simulink model "ErskineMultiDroneFormation"  (R2019b)
settings: Solver=FixedStepAuto  StartTime=0.0  StopTime=Tsim  FixedStep=sim_dt  RelTol=1e-3
values from neighbouring files (symbols this model uses):
  controller_rate = 25    [MultiQuadInit.m]
  drone_params = setDefaultDroneParams(nDrones)    [MultiQuadInit.m]    (also in SingleQuadInit.m = setDefaultDroneParams(1))
  dt_p = 0.1    [MultiQuadInit.m]
  edges = [1,2 ... (first row only)    [MultiQuadInit.m]
  g = 9.81    [MultiQuadInit.m]    (also in SingleQuadInit.m)
  N_p = 1    [MultiQuadInit.m]
  nDrones = 3    [MultiQuadInit.m]
  omega0 = zeros(3,nDrones)    [MultiQuadInit.m]    (also in SingleQuadInit.m = [0;0;0])
  p0 = 4*(rand(3,nDrones) - [0.5;0.5;0])    [MultiQuadInit.m]    (also in SingleQuadInit.m = 4*(rand(3, 1) - [0.5;0.5;0]))
  q0 = zeros(4,nDrones); q0(1,:) = ones(1,nDrones)    [MultiQuadInit.m]    (also in SingleQuadInit.m = [1;0;0;0])
  sim_dt = 0.005    [MultiQuadInit.m]    (also in SingleQuadInit.m)
  v0 = zeros(3, nDrones)    [MultiQuadInit.m]    (also in SingleQuadInit.m = [0;0;0])
undefined symbols (not defined in the file or in its folder): camera_noise
libraries: vrlib x6
(part 1 of 2)
settings Model: Creator=julian  LastModifiedBy=julian

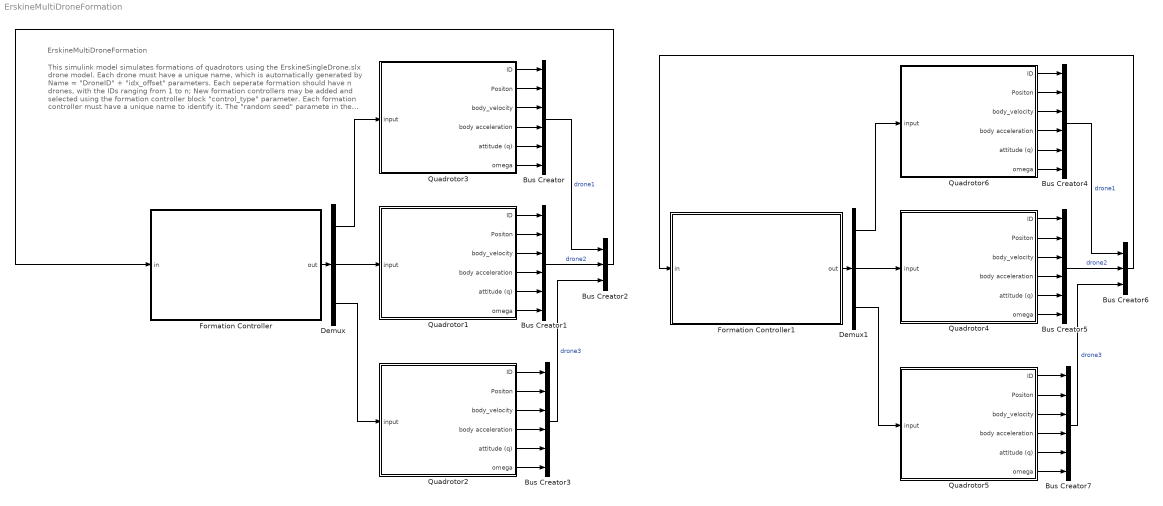
== system ErskineMultiDroneFormation ==
  note: This simulink model simulates formations of quadrotors using the
      | ErskineSingleDrone.slx drone model.  Each drone must have a unique name,
      | which is automatically generated by Name = "DroneID" + "idx_offset" parameters.
      | Each seperate formation should have n drones, with the IDs ranging from 1 to n;
      |
      | New formation controllers may be added and selected using the formation
      | controller block "control_type" parameter. Each formation controller must have a
      | unique name to identify it. The "random seed" paramete in the formation control block sets the random noise seed for the controller measurements.
      |
      | Initial conditions, parameters, and the FormationStateBus must be generated for n drones (see initialization script)
  note: ErskineMultiDroneFormation
  "  Quadrotor1" : Subsystem  mask{control_type_param=2: Body Velocity + Yawrate, DroneID=2, DroneName=Drone2, idx_offset=0}
      mask prompts: control_type_param "Controller type"; DroneName "Drone Name"; idx_offset "Index Offset"
      mask TypeOptions control_type_param: 1: Position + Yaw | 2: Body Velocity + Yawrate | 3: Body Acceleration + Yawrate | 4: Thrust + Attitude | 5: Thrust + Body Rate | 6: Body Wrench
      mask TypeOptions DroneID: 1 | 2 | 3 | 4 | 5 | 6 | 7 | 8 | 9
      mask Callback DroneID:
      | ID = get_param(gcb,'DroneID');
      | offset = get_param(gcb,'idx_offset');
      | if ischar(ID)
      |   ID = str2num(ID);
      | end
      | if ischar(offset)
      |   offset = str2num(offset);
      | end
      | nameID = ID + offset;
      | set_param(gcb,'DroneName',["Drone"+num2str(nameID)]);
      mask Callback DroneName: set_param([gcb,'/To Workspace'],'VariableName',[get_param(gcb,'DroneName')]);
      mask Callback idx_offset:
      | ID = get_param(gcb,'DroneID');
      | offset = get_param(gcb,'idx_offset');
      | if ischar(ID)
      |   ID = str2num(ID);
      | end
      | if ischar(offset)
      |   offset = str2num(offset);
      | end
      | nameID = ID + offset;
      | set_param(gcb,'DroneName',["Drone"+num2str(nameID)]);
      mask DialogControl Control4 Prompt: click to choose controller
      mask Display:
      | image('Format/drone_image.png'); % Use "Edit Image" on toolstrip to change.
      | Name = get_param(gcb,'DroneName');
      | ID = get_param(gcb,'DroneID');
      | C_mode = get_param(gcb,'control_type_param');
      | C_mode(1:2) = [];
      | color('red')
      | ID = "ID = "+ID;
      | color('red')
      | text(0.5, 0.25, Name, 'horizontalAlignment', 'center')
      | color('red')
      | text(0.5, 0.15, ID, 'horizontalAlignment', 'center')
      | color('blue');
      | text(0.5, 0.05, C_mode, 'horizontalAlignment', 'center')
  "  Quadrotor2" : Subsystem  mask{control_type_param=2: Body Velocity + Yawrate, DroneID=3, DroneName=Drone3, idx_offset=0}
      mask prompts: control_type_param "Controller type"; DroneName "Drone Name"; idx_offset "Index Offset"
      mask TypeOptions control_type_param: 1: Position + Yaw | 2: Body Velocity + Yawrate | 3: Body Acceleration + Yawrate | 4: Thrust + Attitude | 5: Thrust + Body Rate | 6: Body Wrench
      mask TypeOptions DroneID: 1 | 2 | 3 | 4 | 5 | 6 | 7 | 8 | 9
      mask Callback DroneID:
      | ID = get_param(gcb,'DroneID');
      | offset = get_param(gcb,'idx_offset');
      | if ischar(ID)
      |   ID = str2num(ID);
      | end
      | if ischar(offset)
      |   offset = str2num(offset);
      | end
      | nameID = ID + offset;
      | set_param(gcb,'DroneName',["Drone"+num2str(nameID)]);
      mask Callback DroneName: set_param([gcb,'/To Workspace'],'VariableName',[get_param(gcb,'DroneName')]);
      mask Callback idx_offset:
      | ID = get_param(gcb,'DroneID');
      | offset = get_param(gcb,'idx_offset');
      | if ischar(ID)
      |   ID = str2num(ID);
      | end
      | if ischar(offset)
      |   offset = str2num(offset);
      | end
      | nameID = ID + offset;
      | set_param(gcb,'DroneName',["Drone"+num2str(nameID)]);
      mask DialogControl Control4 Prompt: click to choose controller
      mask Display:
      | image('Format/drone_image.png'); % Use "Edit Image" on toolstrip to change.
      | Name = get_param(gcb,'DroneName');
      | ID = get_param(gcb,'DroneID');
      | C_mode = get_param(gcb,'control_type_param');
      | C_mode(1:2) = [];
      | color('red')
      | ID = "ID = "+ID;
      | color('red')
      | text(0.5, 0.25, Name, 'horizontalAlignment', 'center')
      | color('red')
      | text(0.5, 0.15, ID, 'horizontalAlignment', 'center')
      | color('blue');
      | text(0.5, 0.05, C_mode, 'horizontalAlignment', 'center')
  "  Quadrotor3" : Subsystem  mask{control_type_param=2: Body Velocity + Yawrate, DroneID=1, DroneName=Drone1, idx_offset=0}
      mask prompts: control_type_param "Controller type"; DroneName "Drone Name"; idx_offset "Index Offset"
      mask TypeOptions control_type_param: 1: Position + Yaw | 2: Body Velocity + Yawrate | 3: Body Acceleration + Yawrate | 4: Thrust + Attitude | 5: Thrust + Body Rate | 6: Body Wrench
      mask TypeOptions DroneID: 1 | 2 | 3 | 4 | 5 | 6 | 7 | 8 | 9
      mask Callback DroneID:
      | ID = get_param(gcb,'DroneID');
      | offset = get_param(gcb,'idx_offset');
      | if ischar(ID)
      |   ID = str2num(ID);
      | end
      | if ischar(offset)
      |   offset = str2num(offset);
      | end
      | nameID = ID + offset;
      | set_param(gcb,'DroneName',["Drone"+num2str(nameID)]);
      mask Callback DroneName: set_param([gcb,'/To Workspace'],'VariableName',[get_param(gcb,'DroneName')]);
      mask Callback idx_offset:
      | ID = get_param(gcb,'DroneID');
      | offset = get_param(gcb,'idx_offset');
      | if ischar(ID)
      |   ID = str2num(ID);
      | end
      | if ischar(offset)
      |   offset = str2num(offset);
      | end
      | nameID = ID + offset;
      | set_param(gcb,'DroneName',["Drone"+num2str(nameID)]);
      mask DialogControl Control4 Prompt: click to choose controller
      mask Display:
      | image('Format/drone_image.png'); % Use "Edit Image" on toolstrip to change.
      | Name = get_param(gcb,'DroneName');
      | ID = get_param(gcb,'DroneID');
      | C_mode = get_param(gcb,'control_type_param');
      | C_mode(1:2) = [];
      | color('red')
      | ID = "ID = "+ID;
      | color('red')
      | text(0.5, 0.25, Name, 'horizontalAlignment', 'center')
      | color('red')
      | text(0.5, 0.15, ID, 'horizontalAlignment', 'center')
      | color('blue');
      | text(0.5, 0.05, C_mode, 'horizontalAlignment', 'center')
  "  Quadrotor4" : Subsystem  mask{control_type_param=2: Body Velocity + Yawrate, DroneID=2, DroneName=Drone5, idx_offset=3}
      mask prompts: control_type_param "Controller type"; DroneName "Drone Name"; idx_offset "Index Offset"
      mask TypeOptions control_type_param: 1: Position + Yaw | 2: Body Velocity + Yawrate | 3: Body Acceleration + Yawrate | 4: Thrust + Attitude | 5: Thrust + Body Rate | 6: Body Wrench
      mask TypeOptions DroneID: 1 | 2 | 3 | 4 | 5 | 6 | 7 | 8 | 9
      mask Callback DroneID:
      | ID = get_param(gcb,'DroneID');
      | offset = get_param(gcb,'idx_offset');
      | if ischar(ID)
      |   ID = str2num(ID);
      | end
      | if ischar(offset)
      |   offset = str2num(offset);
      | end
      | nameID = ID + offset;
      | set_param(gcb,'DroneName',["Drone"+num2str(nameID)]);
      mask Callback DroneName: set_param([gcb,'/To Workspace'],'VariableName',[get_param(gcb,'DroneName')]);
      mask Callback idx_offset:
      | ID = get_param(gcb,'DroneID');
      | offset = get_param(gcb,'idx_offset');
      | if ischar(ID)
      |   ID = str2num(ID);
      | end
      | if ischar(offset)
      |   offset = str2num(offset);
      | end
      | nameID = ID + offset;
      | set_param(gcb,'DroneName',["Drone"+num2str(nameID)]);
      mask DialogControl Control4 Prompt: click to choose controller
      mask Display:
      | image('Format/drone_image.png'); % Use "Edit Image" on toolstrip to change.
      | Name = get_param(gcb,'DroneName');
      | ID = get_param(gcb,'DroneID');
      | C_mode = get_param(gcb,'control_type_param');
      | C_mode(1:2) = [];
      | color('red')
      | ID = "ID = "+ID;
      | color('red')
      | text(0.5, 0.25, Name, 'horizontalAlignment', 'center')
      | color('red')
      | text(0.5, 0.15, ID, 'horizontalAlignment', 'center')
      | color('blue');
      | text(0.5, 0.05, C_mode, 'horizontalAlignment', 'center')
  "  Quadrotor5" : Subsystem  mask{control_type_param=2: Body Velocity + Yawrate, DroneID=3, DroneName=Drone6, idx_offset=3}
      mask prompts: control_type_param "Controller type"; DroneName "Drone Name"; idx_offset "Index Offset"
      mask TypeOptions control_type_param: 1: Position + Yaw | 2: Body Velocity + Yawrate | 3: Body Acceleration + Yawrate | 4: Thrust + Attitude | 5: Thrust + Body Rate | 6: Body Wrench
      mask TypeOptions DroneID: 1 | 2 | 3 | 4 | 5 | 6 | 7 | 8 | 9
      mask Callback DroneID:
      | ID = get_param(gcb,'DroneID');
      | offset = get_param(gcb,'idx_offset');
      | if ischar(ID)
      |   ID = str2num(ID);
      | end
      | if ischar(offset)
      |   offset = str2num(offset);
      | end
      | nameID = ID + offset;
      | set_param(gcb,'DroneName',["Drone"+num2str(nameID)]);
      mask Callback DroneName: set_param([gcb,'/To Workspace'],'VariableName',[get_param(gcb,'DroneName')]);
      mask Callback idx_offset:
      | ID = get_param(gcb,'DroneID');
      | offset = get_param(gcb,'idx_offset');
      | if ischar(ID)
      |   ID = str2num(ID);
      | end
      | if ischar(offset)
      |   offset = str2num(offset);
      | end
      | nameID = ID + offset;
      | set_param(gcb,'DroneName',["Drone"+num2str(nameID)]);
      mask DialogControl Control4 Prompt: click to choose controller
      mask Display:
      | image('Format/drone_image.png'); % Use "Edit Image" on toolstrip to change.
      | Name = get_param(gcb,'DroneName');
      | ID = get_param(gcb,'DroneID');
      | C_mode = get_param(gcb,'control_type_param');
      | C_mode(1:2) = [];
      | color('red')
      | ID = "ID = "+ID;
      | color('red')
      | text(0.5, 0.25, Name, 'horizontalAlignment', 'center')
      | color('red')
      | text(0.5, 0.15, ID, 'horizontalAlignment', 'center')
      | color('blue');
      | text(0.5, 0.05, C_mode, 'horizontalAlignment', 'center')
  "  Quadrotor6" : Subsystem  mask{control_type_param=2: Body Velocity + Yawrate, DroneID=1, DroneName=Drone4, idx_offset=3}
      mask prompts: control_type_param "Controller type"; DroneName "Drone Name"; idx_offset "Index Offset"
      mask TypeOptions control_type_param: 1: Position + Yaw | 2: Body Velocity + Yawrate | 3: Body Acceleration + Yawrate | 4: Thrust + Attitude | 5: Thrust + Body Rate | 6: Body Wrench
      mask TypeOptions DroneID: 1 | 2 | 3 | 4 | 5 | 6 | 7 | 8 | 9
      mask Callback DroneID:
      | ID = get_param(gcb,'DroneID');
      | offset = get_param(gcb,'idx_offset');
      | if ischar(ID)
      |   ID = str2num(ID);
      | end
      | if ischar(offset)
      |   offset = str2num(offset);
      | end
      | nameID = ID + offset;
      | set_param(gcb,'DroneName',["Drone"+num2str(nameID)]);
      mask Callback DroneName: set_param([gcb,'/To Workspace'],'VariableName',[get_param(gcb,'DroneName')]);
      mask Callback idx_offset:
      | ID = get_param(gcb,'DroneID');
      | offset = get_param(gcb,'idx_offset');
      | if ischar(ID)
      |   ID = str2num(ID);
      | end
      | if ischar(offset)
      |   offset = str2num(offset);
      | end
      | nameID = ID + offset;
      | set_param(gcb,'DroneName',["Drone"+num2str(nameID)]);
      mask DialogControl Control4 Prompt: click to choose controller
      mask Display:
      | image('Format/drone_image.png'); % Use "Edit Image" on toolstrip to change.
      | Name = get_param(gcb,'DroneName');
      | ID = get_param(gcb,'DroneID');
      | C_mode = get_param(gcb,'control_type_param');
      | C_mode(1:2) = [];
      | color('red')
      | ID = "ID = "+ID;
      | color('red')
      | text(0.5, 0.25, Name, 'horizontalAlignment', 'center')
      | color('red')
      | text(0.5, 0.15, ID, 'horizontalAlignment', 'center')
      | color('blue');
      | text(0.5, 0.05, C_mode, 'horizontalAlignment', 'center')
  Bus Creator{,1,3..5,7} (6 alike) : BusCreator  Inputs=6  OutDataTypeStr=Bus: DroneStateBus
      settings: InheritFromInputs=off
  Bus Creator2 : BusCreator  Inputs=3  OutDataTypeStr=Bus: FormationStateBus  NonVirtualBus=on
      settings: InheritFromInputs=off
  Bus Creator6 : BusCreator  Inputs=3  OutDataTypeStr=Bus: FormationStateBus  NonVirtualBus=on
      settings: InheritFromInputs=off
  Demux : Demux  Outputs=3
  Demux1 : Demux  Outputs=3
  Formation Controller : Subsystem  mask(FormationController){seed_type=Random, rng_seed=9730, control_type=1: Gradient, out_name=Gradient}
      mask prompts: seed_type "Random Seed"; rng_seed "Custom Seed"; control_type "Formation Control Type"; out_name "Out Name"
      mask TypeOptions seed_type: Random | Custom
      mask Callback seed_type:
      | box_A = get_param(gcb, 'seed_type');
      | m = Simulink.Mask.get(gcb);
      | box_B = m.getParameter('rng_seed');
      | 
      | if strcmp(box_A, 'Random')
      |     seed = randi([1,10000]);
      |     set_param(gcb,'rng_seed', num2str(seed));
      |     box_B.Enabled = 'off';
      | else
      |     box_B.Enabled = 'on';
      | end
      mask TypeOptions control_type: 1: Gradient | 2: Faster Gradient
      mask Callback out_name: set_param([gcb,'/To Workspace'],'VariableName',[get_param(gcb,'out_name')]);
      mask Display:
      | image('$imagefile'); % Use "Edit Image" on toolstrip to change.
      | type = get_param(gcb,'control_type');
      | color('red')
      | text(0.5, 0.25, type, 'horizontalAlignment', 'center')
  Formation Controller1 : Subsystem  mask(FormationController){seed_type=Random, rng_seed=5186, control_type=2: Faster Gradient, out_name=PoorlyTunedGradient}
      mask prompts: seed_type "Random Seed"; rng_seed "Custom Seed"; control_type "Formation Control Type"; out_name "Out Name"
      mask TypeOptions seed_type: Random | Custom
      mask Callback seed_type:
      | box_A = get_param(gcb, 'seed_type');
      | m = Simulink.Mask.get(gcb);
      | box_B = m.getParameter('rng_seed');
      | 
      | if strcmp(box_A, 'Random')
      |     seed = randi([1,10000]);
      |     set_param(gcb,'rng_seed', num2str(seed));
      |     box_B.Enabled = 'off';
      | else
      |     box_B.Enabled = 'on';
      | end
      mask TypeOptions control_type: 1: Gradient | 2: Faster Gradient
      mask Callback out_name: set_param([gcb,'/To Workspace'],'VariableName',[get_param(gcb,'out_name')]);
      mask Display:
      | image('$imagefile'); % Use "Edit Image" on toolstrip to change.
      | type = get_param(gcb,'control_type');
      | color('red')
      | text(0.5, 0.25, type, 'horizontalAlignment', 'center')
  wires:
  "  Quadrotor3"/6(omega) -> Bus Creator/6
  "  Quadrotor3"/5(attitude (q)) -> Bus Creator/5
  "  Quadrotor3"/4(body acceleration) -> Bus Creator/4
  "  Quadrotor3"/3(body_velocity) -> Bus Creator/3
  "  Quadrotor3"/2(Positon) -> Bus Creator/2
  "  Quadrotor3"/1(ID) -> Bus Creator/1
  "  Quadrotor1"/1(ID) -> Bus Creator1/1
  "  Quadrotor1"/2(Positon) -> Bus Creator1/2
  "  Quadrotor1"/3(body_velocity) -> Bus Creator1/3
  "  Quadrotor1"/4(body acceleration) -> Bus Creator1/4
  "  Quadrotor1"/5(attitude (q)) -> Bus Creator1/5
  "  Quadrotor1"/6(omega) -> Bus Creator1/6
  Bus Creator/1 -> Bus Creator2/1  "drone1"
  Bus Creator1/1 -> Bus Creator2/2  "drone2"
  Bus Creator2/1 -> Formation Controller/1(in)
  Formation Controller/1(out) -> Demux/1
  "  Quadrotor2"/1(ID) -> Bus Creator3/1
  "  Quadrotor2"/2(Positon) -> Bus Creator3/2
  "  Quadrotor2"/3(body_velocity) -> Bus Creator3/3
  "  Quadrotor2"/4(body acceleration) -> Bus Creator3/4
  "  Quadrotor2"/5(attitude (q)) -> Bus Creator3/5
  "  Quadrotor2"/6(omega) -> Bus Creator3/6
  Bus Creator3/1 -> Bus Creator2/3  "drone3"
  Demux/1 -> "  Quadrotor3"/1(input)
  Demux/2 -> "  Quadrotor1"/1(input)
  Demux/3 -> "  Quadrotor2"/1(input)
  Demux1/2 -> "  Quadrotor4"/1(input)
  "  Quadrotor5"/3(body_velocity) -> Bus Creator7/3
  "  Quadrotor6"/1(ID) -> Bus Creator4/1
  "  Quadrotor6"/4(body acceleration) -> Bus Creator4/4
  "  Quadrotor4"/1(ID) -> Bus Creator5/1
  "  Quadrotor4"/2(Positon) -> Bus Creator5/2
  "  Quadrotor6"/2(Positon) -> Bus Creator4/2
  "  Quadrotor4"/3(body_velocity) -> Bus Creator5/3
  "  Quadrotor4"/4(body acceleration) -> Bus Creator5/4
  "  Quadrotor4"/5(attitude (q)) -> Bus Creator5/5
  "  Quadrotor6"/6(omega) -> Bus Creator4/6
  Bus Creator6/1 -> Formation Controller1/1(in)
  "  Quadrotor5"/4(body acceleration) -> Bus Creator7/4
  Bus Creator4/1 -> Bus Creator6/1  "drone1"
  "  Quadrotor4"/6(omega) -> Bus Creator5/6
  Bus Creator5/1 -> Bus Creator6/2  "drone2"
  "  Quadrotor5"/2(Positon) -> Bus Creator7/2
  Demux1/1 -> "  Quadrotor6"/1(input)
  Bus Creator7/1 -> Bus Creator6/3  "drone3"
  Formation Controller1/1(out) -> Demux1/1
  "  Quadrotor5"/6(omega) -> Bus Creator7/6
  "  Quadrotor6"/5(attitude (q)) -> Bus Creator4/5
  Demux1/3 -> "  Quadrotor5"/1(input)
  "  Quadrotor6"/3(body_velocity) -> Bus Creator4/3
  "  Quadrotor5"/5(attitude (q)) -> Bus Creator7/5
  "  Quadrotor5"/1(ID) -> Bus Creator7/1

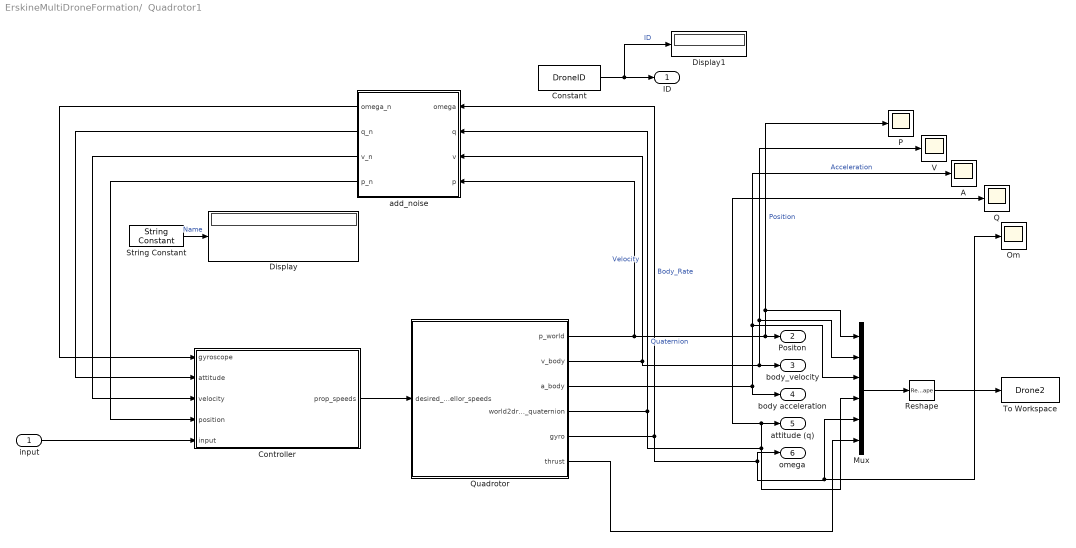
== system ErskineMultiDroneFormation/  Quadrotor1 ==
  input : Inport
  A : Scope
  Constant : Constant  Value=DroneID
  Controller : Subsystem
      mask Display: image('Format/flightController.png'); % Use "Edit Image" on toolstrip to change.
  Display : Display
  Display1 : Display
  Mux : Mux  Inputs=6
  Om : Scope
  P : Scope
  Q : Scope
  Quadrotor : Subsystem
      mask Display: image('droneHardware.jpeg'); % Use "Edit Image" on toolstrip to change.
  Reshape : Reshape
  String Constant : StringConstant  String=DroneName
  To Workspace : ToWorkspace  VariableName=Drone2  SaveFormat=Timeseries  SampleTime=-1
  V : Scope
  add_noise : MATLAB Function  TreatAsAtomicUnit=on
  ID : Outport
  Positon : Outport  Port=2
  body_velocity : Outport  Port=3
  body acceleration : Outport  Port=4
  attitude (q) : Outport  Port=5
  omega : Outport  Port=6
  wires:
  Quadrotor/5(gyro) -> Om/1, Mux/5, omega/1, add_noise/1(omega)  "Body_Rate"
  Quadrotor/1(p_world) -> add_noise/4(p), P/1, Mux/1, Positon/1  "Position"
  Quadrotor/3(a_body) -> body acceleration/1, A/1, Mux/3  "Acceleration"
  Quadrotor/4(world2drone_quaternion) -> Q/1, attitude (q)/1, Mux/4, add_noise/2(q)  "Quaternion"
  Mux/1 -> Reshape/1
  Quadrotor/2(v_body) -> V/1, Mux/2, body_velocity/1, add_noise/3(v)  "Velocity"
  Quadrotor/6(thrust) -> Mux/6
  String Constant/1 -> Display/1  "Name"
  Constant/1 -> Display1/1, ID/1  "ID"
  Reshape/1 -> To Workspace/1
  add_noise/1(omega_n) -> Controller/1(gyroscope)
  add_noise/2(q_n) -> Controller/2(attitude)
  add_noise/3(v_n) -> Controller/3(velocity)
  add_noise/4(p_n) -> Controller/4(position)
  input/1 -> Controller/5(input)
  Controller/1(prop_speeds) -> Quadrotor/1(desired_propellor_speeds)

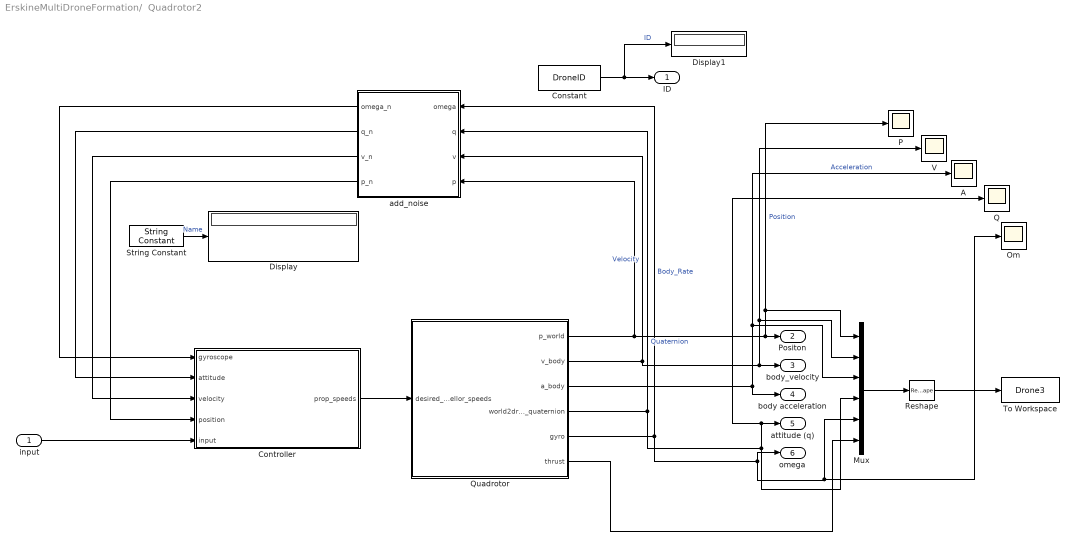
== system ErskineMultiDroneFormation/  Quadrotor2 ==
  input : Inport
  A : Scope
  Constant : Constant  Value=DroneID
  Controller : Subsystem
      mask Display: image('Format/flightController.png'); % Use "Edit Image" on toolstrip to change.
  Display : Display
  Display1 : Display
  Mux : Mux  Inputs=6
  Om : Scope
  P : Scope
  Q : Scope
  Quadrotor : Subsystem
      mask Display: image('droneHardware.jpeg'); % Use "Edit Image" on toolstrip to change.
  Reshape : Reshape
  String Constant : StringConstant  String=DroneName
  To Workspace : ToWorkspace  VariableName=Drone3  SaveFormat=Timeseries  SampleTime=-1
  V : Scope
  add_noise : MATLAB Function  TreatAsAtomicUnit=on
  ID : Outport
  Positon : Outport  Port=2
  body_velocity : Outport  Port=3
  body acceleration : Outport  Port=4
  attitude (q) : Outport  Port=5
  omega : Outport  Port=6
  wires:
  Quadrotor/5(gyro) -> Om/1, Mux/5, omega/1, add_noise/1(omega)  "Body_Rate"
  Quadrotor/1(p_world) -> add_noise/4(p), P/1, Mux/1, Positon/1  "Position"
  Quadrotor/3(a_body) -> body acceleration/1, A/1, Mux/3  "Acceleration"
  Quadrotor/4(world2drone_quaternion) -> Q/1, attitude (q)/1, Mux/4, add_noise/2(q)  "Quaternion"
  Mux/1 -> Reshape/1
  Quadrotor/2(v_body) -> V/1, Mux/2, body_velocity/1, add_noise/3(v)  "Velocity"
  Quadrotor/6(thrust) -> Mux/6
  String Constant/1 -> Display/1  "Name"
  Constant/1 -> Display1/1, ID/1  "ID"
  Reshape/1 -> To Workspace/1
  add_noise/1(omega_n) -> Controller/1(gyroscope)
  add_noise/2(q_n) -> Controller/2(attitude)
  add_noise/3(v_n) -> Controller/3(velocity)
  add_noise/4(p_n) -> Controller/4(position)
  input/1 -> Controller/5(input)
  Controller/1(prop_speeds) -> Quadrotor/1(desired_propellor_speeds)

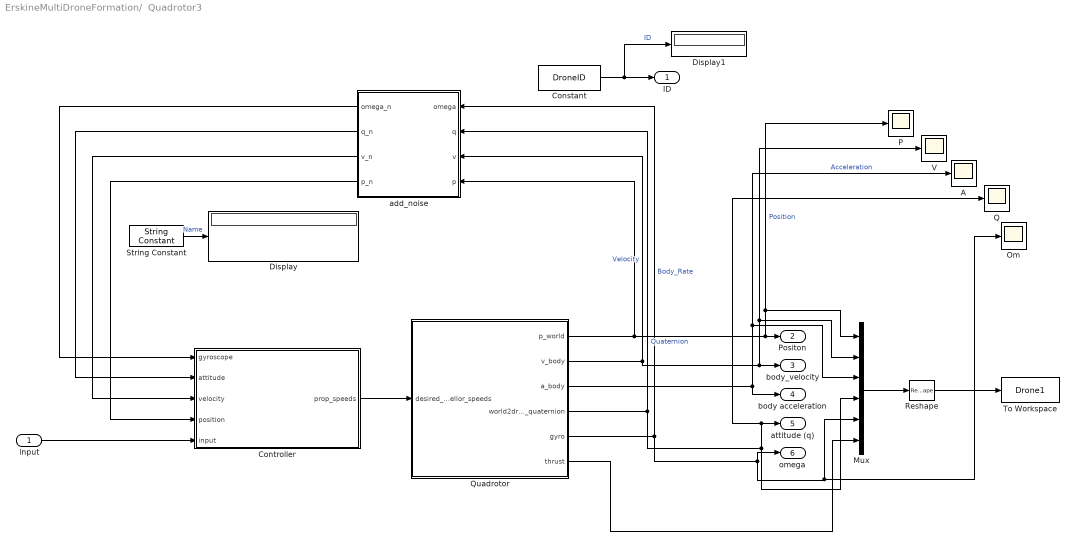
== system ErskineMultiDroneFormation/  Quadrotor3 ==
  input : Inport
  A : Scope
  Constant : Constant  Value=DroneID
  Controller : Subsystem
      mask Display: image('Format/flightController.png'); % Use "Edit Image" on toolstrip to change.
  Display : Display
  Display1 : Display
  Mux : Mux  Inputs=6
  Om : Scope
  P : Scope
  Q : Scope
  Quadrotor : Subsystem
      mask Display: image('droneHardware.jpeg'); % Use "Edit Image" on toolstrip to change.
  Reshape : Reshape
  String Constant : StringConstant  String=DroneName
  To Workspace : ToWorkspace  VariableName=Drone1  SaveFormat=Timeseries  SampleTime=-1
  V : Scope
  add_noise : MATLAB Function  TreatAsAtomicUnit=on
  ID : Outport
  Positon : Outport  Port=2
  body_velocity : Outport  Port=3
  body acceleration : Outport  Port=4
  attitude (q) : Outport  Port=5
  omega : Outport  Port=6
  wires:
  Quadrotor/5(gyro) -> Om/1, Mux/5, omega/1, add_noise/1(omega)  "Body_Rate"
  Quadrotor/1(p_world) -> add_noise/4(p), P/1, Mux/1, Positon/1  "Position"
  Quadrotor/3(a_body) -> body acceleration/1, A/1, Mux/3  "Acceleration"
  Quadrotor/4(world2drone_quaternion) -> Q/1, attitude (q)/1, Mux/4, add_noise/2(q)  "Quaternion"
  Mux/1 -> Reshape/1
  Quadrotor/2(v_body) -> V/1, Mux/2, body_velocity/1, add_noise/3(v)  "Velocity"
  Quadrotor/6(thrust) -> Mux/6
  String Constant/1 -> Display/1  "Name"
  Constant/1 -> Display1/1, ID/1  "ID"
  Reshape/1 -> To Workspace/1
  add_noise/1(omega_n) -> Controller/1(gyroscope)
  add_noise/2(q_n) -> Controller/2(attitude)
  add_noise/3(v_n) -> Controller/3(velocity)
  add_noise/4(p_n) -> Controller/4(position)
  input/1 -> Controller/5(input)
  Controller/1(prop_speeds) -> Quadrotor/1(desired_propellor_speeds)

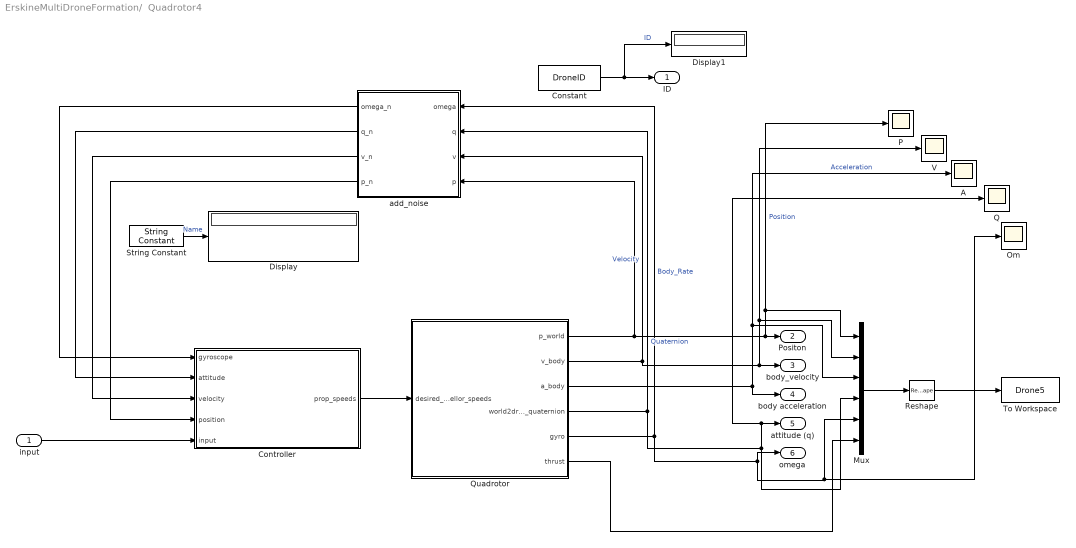
== system ErskineMultiDroneFormation/  Quadrotor4 ==
  input : Inport
  A : Scope
  Constant : Constant  Value=DroneID
  Controller : Subsystem
      mask Display: image('Format/flightController.png'); % Use "Edit Image" on toolstrip to change.
  Display : Display
  Display1 : Display
  Mux : Mux  Inputs=6
  Om : Scope
  P : Scope
  Q : Scope
  Quadrotor : Subsystem
      mask Display: image('droneHardware.jpeg'); % Use "Edit Image" on toolstrip to change.
  Reshape : Reshape
  String Constant : StringConstant  String=DroneName
  To Workspace : ToWorkspace  VariableName=Drone5  SaveFormat=Timeseries  SampleTime=-1
  V : Scope
  add_noise : MATLAB Function  TreatAsAtomicUnit=on
  ID : Outport
  Positon : Outport  Port=2
  body_velocity : Outport  Port=3
  body acceleration : Outport  Port=4
  attitude (q) : Outport  Port=5
  omega : Outport  Port=6
  wires:
  Quadrotor/5(gyro) -> Om/1, Mux/5, omega/1, add_noise/1(omega)  "Body_Rate"
  Quadrotor/1(p_world) -> add_noise/4(p), P/1, Mux/1, Positon/1  "Position"
  Quadrotor/3(a_body) -> body acceleration/1, A/1, Mux/3  "Acceleration"
  Quadrotor/4(world2drone_quaternion) -> Q/1, attitude (q)/1, Mux/4, add_noise/2(q)  "Quaternion"
  Mux/1 -> Reshape/1
  Quadrotor/2(v_body) -> V/1, Mux/2, body_velocity/1, add_noise/3(v)  "Velocity"
  Quadrotor/6(thrust) -> Mux/6
  String Constant/1 -> Display/1  "Name"
  Constant/1 -> Display1/1, ID/1  "ID"
  Reshape/1 -> To Workspace/1
  add_noise/1(omega_n) -> Controller/1(gyroscope)
  add_noise/2(q_n) -> Controller/2(attitude)
  add_noise/3(v_n) -> Controller/3(velocity)
  add_noise/4(p_n) -> Controller/4(position)
  input/1 -> Controller/5(input)
  Controller/1(prop_speeds) -> Quadrotor/1(desired_propellor_speeds)

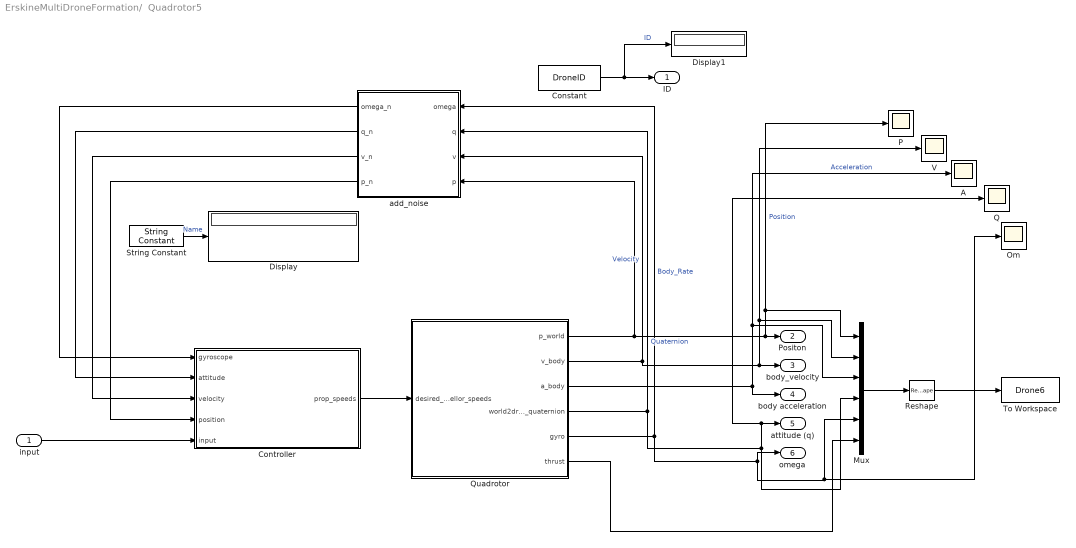
== system ErskineMultiDroneFormation/  Quadrotor5 ==
  input : Inport
  A : Scope
  Constant : Constant  Value=DroneID
  Controller : Subsystem
      mask Display: image('Format/flightController.png'); % Use "Edit Image" on toolstrip to change.
  Display : Display
  Display1 : Display
  Mux : Mux  Inputs=6
  Om : Scope
  P : Scope
  Q : Scope
  Quadrotor : Subsystem
      mask Display: image('droneHardware.jpeg'); % Use "Edit Image" on toolstrip to change.
  Reshape : Reshape
  String Constant : StringConstant  String=DroneName
  To Workspace : ToWorkspace  VariableName=Drone6  SaveFormat=Timeseries  SampleTime=-1
  V : Scope
  add_noise : MATLAB Function  TreatAsAtomicUnit=on
  ID : Outport
  Positon : Outport  Port=2
  body_velocity : Outport  Port=3
  body acceleration : Outport  Port=4
  attitude (q) : Outport  Port=5
  omega : Outport  Port=6
  wires:
  Quadrotor/5(gyro) -> Om/1, Mux/5, omega/1, add_noise/1(omega)  "Body_Rate"
  Quadrotor/1(p_world) -> add_noise/4(p), P/1, Mux/1, Positon/1  "Position"
  Quadrotor/3(a_body) -> body acceleration/1, A/1, Mux/3  "Acceleration"
  Quadrotor/4(world2drone_quaternion) -> Q/1, attitude (q)/1, Mux/4, add_noise/2(q)  "Quaternion"
  Mux/1 -> Reshape/1
  Quadrotor/2(v_body) -> V/1, Mux/2, body_velocity/1, add_noise/3(v)  "Velocity"
  Quadrotor/6(thrust) -> Mux/6
  String Constant/1 -> Display/1  "Name"
  Constant/1 -> Display1/1, ID/1  "ID"
  Reshape/1 -> To Workspace/1
  add_noise/1(omega_n) -> Controller/1(gyroscope)
  add_noise/2(q_n) -> Controller/2(attitude)
  add_noise/3(v_n) -> Controller/3(velocity)
  add_noise/4(p_n) -> Controller/4(position)
  input/1 -> Controller/5(input)
  Controller/1(prop_speeds) -> Quadrotor/1(desired_propellor_speeds)

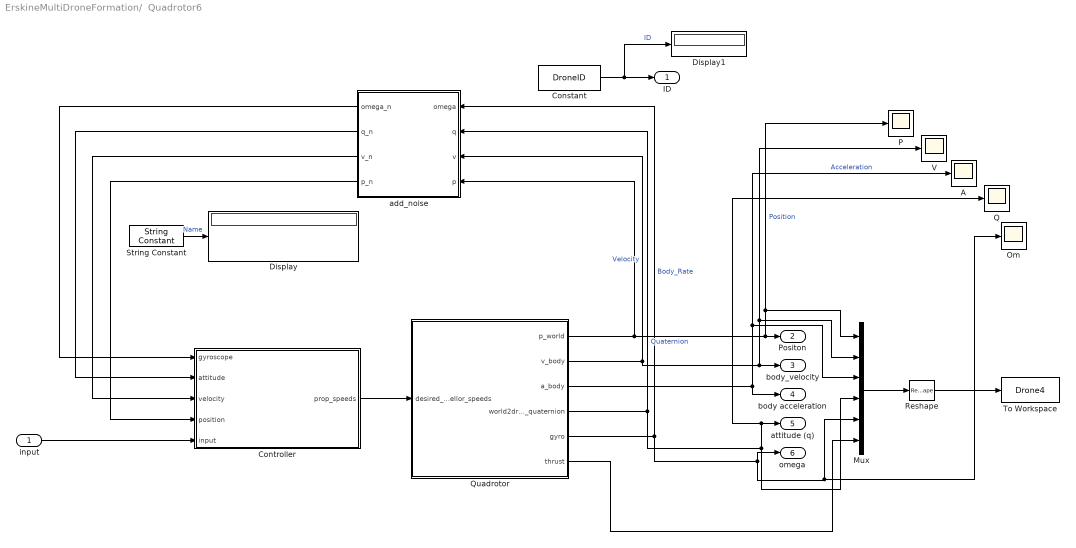
== system ErskineMultiDroneFormation/  Quadrotor6 ==
  input : Inport
  A : Scope
  Constant : Constant  Value=DroneID
  Controller : Subsystem
      mask Display: image('Format/flightController.png'); % Use "Edit Image" on toolstrip to change.
  Display : Display
  Display1 : Display
  Mux : Mux  Inputs=6
  Om : Scope
  P : Scope
  Q : Scope
  Quadrotor : Subsystem
      mask Display: image('droneHardware.jpeg'); % Use "Edit Image" on toolstrip to change.
  Reshape : Reshape
  String Constant : StringConstant  String=DroneName
  To Workspace : ToWorkspace  VariableName=Drone4  SaveFormat=Timeseries  SampleTime=-1
  V : Scope
  add_noise : MATLAB Function  TreatAsAtomicUnit=on
  ID : Outport
  Positon : Outport  Port=2
  body_velocity : Outport  Port=3
  body acceleration : Outport  Port=4
  attitude (q) : Outport  Port=5
  omega : Outport  Port=6
  wires:
  Quadrotor/5(gyro) -> Om/1, Mux/5, omega/1, add_noise/1(omega)  "Body_Rate"
  Quadrotor/1(p_world) -> add_noise/4(p), P/1, Mux/1, Positon/1  "Position"
  Quadrotor/3(a_body) -> body acceleration/1, A/1, Mux/3  "Acceleration"
  Quadrotor/4(world2drone_quaternion) -> Q/1, attitude (q)/1, Mux/4, add_noise/2(q)  "Quaternion"
  Mux/1 -> Reshape/1
  Quadrotor/2(v_body) -> V/1, Mux/2, body_velocity/1, add_noise/3(v)  "Velocity"
  Quadrotor/6(thrust) -> Mux/6
  String Constant/1 -> Display/1  "Name"
  Constant/1 -> Display1/1, ID/1  "ID"
  Reshape/1 -> To Workspace/1
  add_noise/1(omega_n) -> Controller/1(gyroscope)
  add_noise/2(q_n) -> Controller/2(attitude)
  add_noise/3(v_n) -> Controller/3(velocity)
  add_noise/4(p_n) -> Controller/4(position)
  input/1 -> Controller/5(input)
  Controller/1(prop_speeds) -> Quadrotor/1(desired_propellor_speeds)

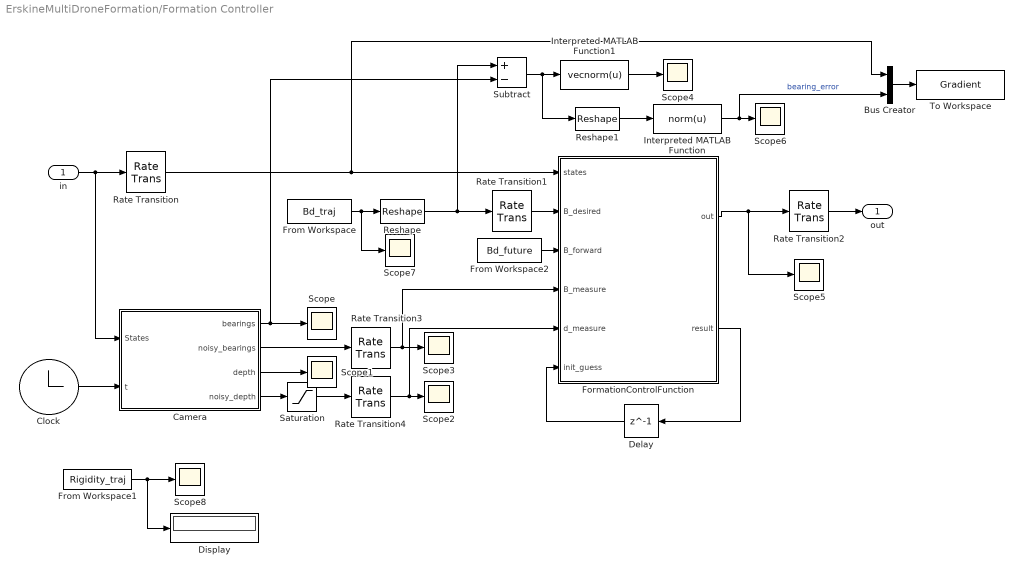
== system ErskineMultiDroneFormation/Formation Controller ==
  in : Inport
  Bus Creator : BusCreator  Inputs=2
  Camera : MATLAB Function  TreatAsAtomicUnit=on  SystemSampleTime=sim_dt
  Clock : Clock
  Delay : Delay  DelayLength=1  InitialCondition=zeros(nDrones*4*N_p, 1)
  Display : Display
  FormationControlFunction : MATLAB Function  TreatAsAtomicUnit=on
  From Workspace : FromWorkspace  VariableName=Bd_traj  SampleTime=sim_dt  OutputAfterFinalValue=Holding final value
  From Workspace1 : FromWorkspace  VariableName=Rigidity_traj  SampleTime=sim_dt  OutputAfterFinalValue=Holding final value
  From Workspace2 : FromWorkspace  VariableName=Bd_future  SampleTime=sim_dt  OutputAfterFinalValue=Holding final value
  Interpreted MATLAB Function : MATLABFcn  MATLABFcn=norm(u)
  Interpreted MATLAB Function1 : MATLABFcn  MATLABFcn=vecnorm(u)
  Rate Transition{,1,3..4} (4 alike) : RateTransition  OutPortSampleTime=1/controller_rate
  Rate Transition2 : RateTransition  OutPortSampleTime=sim_dt
  Reshape : Reshape  OutputDimensionality=Customize  OutputDimensions=[3,length(edges)]
  Reshape1 : Reshape  OutputDimensions=[3,length(edges)]
  Saturation : Saturate  UpperLimit=999999  LowerLimit=0.2
  Scope{,1..8} (9 alike) : Scope
  Subtract : Sum  Inputs=+-
  To Workspace : ToWorkspace  VariableName=Gradient  SaveFormat=Timeseries  SampleTime=-1
  out : Outport
  wires:
  in/1 -> Camera/1(States), Rate Transition/1
  FormationControlFunction/1(out) -> Scope5/1, Rate Transition2/1
  FormationControlFunction/2(result) -> Delay/1
  Delay/1 -> FormationControlFunction/6(init_guess)
  Camera/1(bearings) -> Scope/1, Subtract/2
  Rate Transition/1 -> Bus Creator/1, FormationControlFunction/1(states)
  Rate Transition1/1 -> FormationControlFunction/2(B_desired)
  Rate Transition2/1 -> out/1
  Camera/3(depth) -> Scope1/1
  Camera/4(noisy_depth) -> Saturation/1
  Camera/2(noisy_bearings) -> Rate Transition3/1
  Rate Transition3/1 -> FormationControlFunction/4(B_measure), Scope3/1
  Rate Transition4/1 -> FormationControlFunction/5(d_measure), Scope2/1
  Reshape/1 -> Rate Transition1/1, Subtract/1
  Subtract/1 -> Reshape1/1, Interpreted MATLAB Function1/1
  Interpreted MATLAB Function/1 -> Bus Creator/2, Scope6/1  "bearing_error"
  Reshape1/1 -> Interpreted MATLAB Function/1
  Saturation/1 -> Rate Transition4/1
  From Workspace/1 -> Scope7/1, Reshape/1
  Clock/1 -> Camera/2(t)
  Interpreted MATLAB Function1/1 -> Scope4/1
  From Workspace1/1 -> Display/1, Scope8/1
  From Workspace2/1 -> FormationControlFunction/3(B_forward)
  Bus Creator/1 -> To Workspace/1

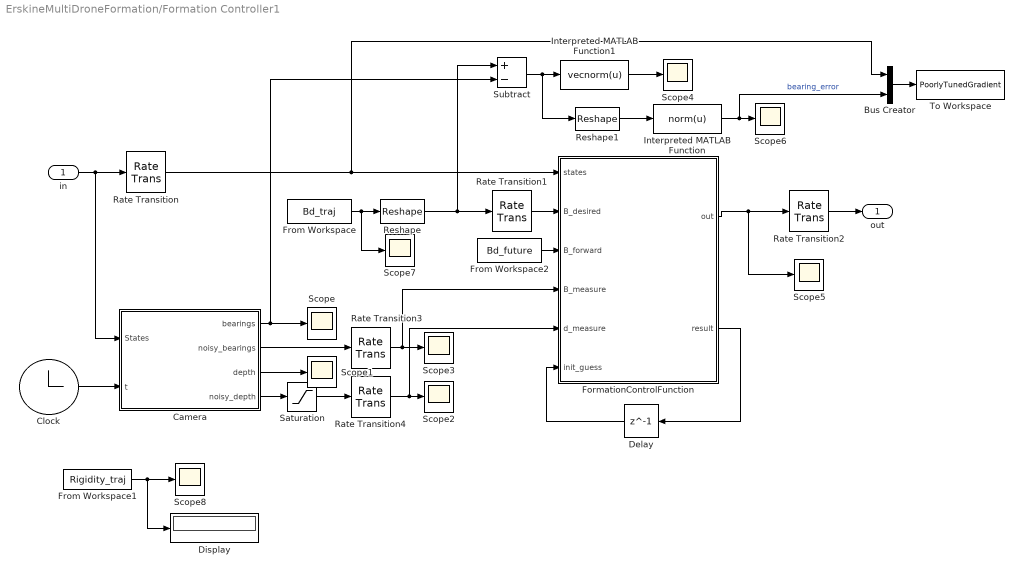
== system ErskineMultiDroneFormation/Formation Controller1 ==
  in : Inport
  Bus Creator : BusCreator  Inputs=2
  Camera : MATLAB Function  TreatAsAtomicUnit=on  SystemSampleTime=sim_dt
  Clock : Clock
  Delay : Delay  DelayLength=1  InitialCondition=zeros(nDrones*4*N_p, 1)
  Display : Display
  FormationControlFunction : MATLAB Function  TreatAsAtomicUnit=on
  From Workspace : FromWorkspace  VariableName=Bd_traj  SampleTime=sim_dt  OutputAfterFinalValue=Holding final value
  From Workspace1 : FromWorkspace  VariableName=Rigidity_traj  SampleTime=sim_dt  OutputAfterFinalValue=Holding final value
  From Workspace2 : FromWorkspace  VariableName=Bd_future  SampleTime=sim_dt  OutputAfterFinalValue=Holding final value
  Interpreted MATLAB Function : MATLABFcn  MATLABFcn=norm(u)
  Interpreted MATLAB Function1 : MATLABFcn  MATLABFcn=vecnorm(u)
  Rate Transition{,1,3..4} (4 alike) : RateTransition  OutPortSampleTime=1/controller_rate
  Rate Transition2 : RateTransition  OutPortSampleTime=sim_dt
  Reshape : Reshape  OutputDimensionality=Customize  OutputDimensions=[3,length(edges)]
  Reshape1 : Reshape  OutputDimensions=[3,length(edges)]
  Saturation : Saturate  UpperLimit=999999  LowerLimit=0.2
  Scope{,1..8} (9 alike) : Scope
  Subtract : Sum  Inputs=+-
  To Workspace : ToWorkspace  VariableName=PoorlyTunedGradient  SaveFormat=Timeseries  SampleTime=-1
  out : Outport
  wires:
  in/1 -> Camera/1(States), Rate Transition/1
  FormationControlFunction/1(out) -> Scope5/1, Rate Transition2/1
  FormationControlFunction/2(result) -> Delay/1
  Delay/1 -> FormationControlFunction/6(init_guess)
  Camera/1(bearings) -> Scope/1, Subtract/2
  Rate Transition/1 -> Bus Creator/1, FormationControlFunction/1(states)
  Rate Transition1/1 -> FormationControlFunction/2(B_desired)
  Rate Transition2/1 -> out/1
  Camera/3(depth) -> Scope1/1
  Camera/4(noisy_depth) -> Saturation/1
  Camera/2(noisy_bearings) -> Rate Transition3/1
  Rate Transition3/1 -> FormationControlFunction/4(B_measure), Scope3/1
  Rate Transition4/1 -> FormationControlFunction/5(d_measure), Scope2/1
  Reshape/1 -> Rate Transition1/1, Subtract/1
  Subtract/1 -> Reshape1/1, Interpreted MATLAB Function1/1
  Interpreted MATLAB Function/1 -> Bus Creator/2, Scope6/1  "bearing_error"
  Reshape1/1 -> Interpreted MATLAB Function/1
  Saturation/1 -> Rate Transition4/1
  From Workspace/1 -> Scope7/1, Reshape/1
  Clock/1 -> Camera/2(t)
  Interpreted MATLAB Function1/1 -> Scope4/1
  From Workspace1/1 -> Display/1, Scope8/1
  From Workspace2/1 -> FormationControlFunction/3(B_forward)
  Bus Creator/1 -> To Workspace/1

== system ErskineMultiDroneFormation/  Quadrotor1/Controller ==
  gyroscope : Inport
  attitude : Inport  Port=2
  velocity : Inport  Port=3
  position : Inport  Port=4
  input : Inport  Port=5
  Controller : MATLAB Function  TreatAsAtomicUnit=on
  Saturation : Saturate  UpperLimit=drone_params(DroneID).control.limits.thrust.max  LowerLimit=drone_params(DroneID).control.limits.thrust.min
  Saturation1 : Saturate  UpperLimit=0.1  LowerLimit=-0.1
  desired_prop_speed : MATLAB Function  TreatAsAtomicUnit=on
  prop_speeds : Outport
  wires:
  Controller/2(moments) -> Saturation1/1
  Saturation/1 -> desired_prop_speed/1(thrust)
  velocity/1 -> Controller/3(v)
  Saturation1/1 -> desired_prop_speed/2(moment)
  Controller/1(thrust) -> Saturation/1
  position/1 -> Controller/2(p)
  input/1 -> Controller/1(u)
  attitude/1 -> Controller/4(q)
  gyroscope/1 -> Controller/5(omega)
  desired_prop_speed/1(Omega_props) -> prop_speeds/1

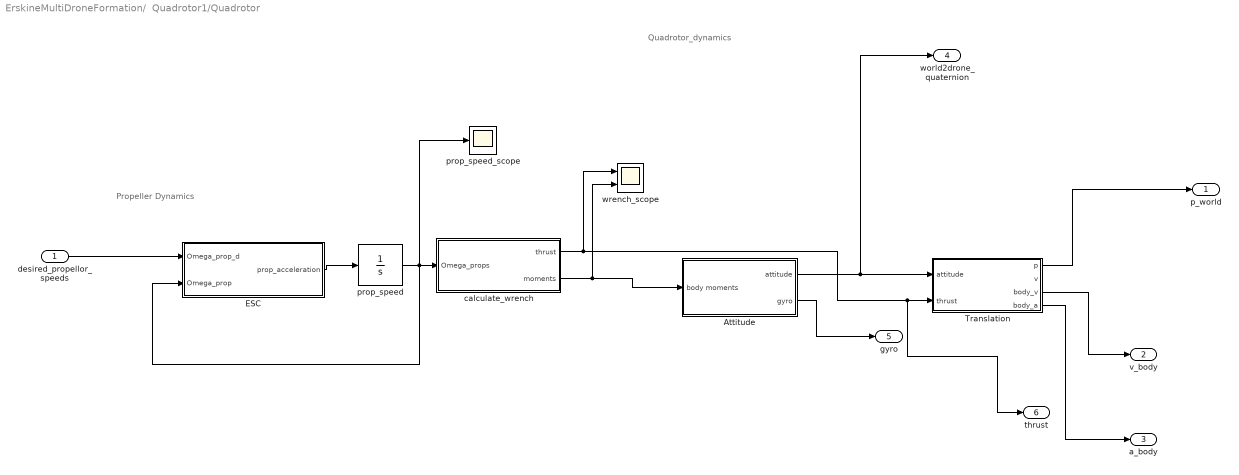
== system ErskineMultiDroneFormation/  Quadrotor1/Quadrotor ==
  note: Quadrotor_dynamics
  note: Propeller Dynamics
  desired_propellor_speeds : Inport
  Attitude : Subsystem
  ESC : MATLAB Function  TreatAsAtomicUnit=on
  Translation : Subsystem
  calculate_wrench : MATLAB Function  TreatAsAtomicUnit=on
  prop_speed : Integrator  InitialCondition=drone_params(DroneID).motors.omega0  LimitOutput=on  UpperSaturationLimit=drone_params(DroneID).motors.omega_max  LowerSaturationLimit=drone_params(DroneID).motors.omega_min
  prop_speed_scope : Scope
  wrench_scope : Scope  NumInputPorts=2
  p_world : Outport
  v_body : Outport  Port=2
  a_body : Outport  Port=3
  world2drone_quaternion : Outport  Port=4
  gyro : Outport  Port=5
  thrust : Outport  Port=6
  wires:
  calculate_wrench/1(thrust) -> wrench_scope/1, thrust/1, Translation/2(thrust)
  ESC/1(prop_acceleration) -> prop_speed/1
  desired_propellor_speeds/1 -> ESC/1(Omega_prop_d)
  prop_speed/1 -> prop_speed_scope/1, calculate_wrench/1(Omega_props), ESC/2(Omega_prop)
  calculate_wrench/2(moments) -> wrench_scope/2, Attitude/1(body moments)
  Attitude/1(attitude) -> world2drone_quaternion/1, Translation/1(attitude)
  Attitude/2(gyro) -> gyro/1
  Translation/3(body_v) -> v_body/1
  Translation/4(body_a) -> a_body/1
  Translation/1(p) -> p_world/1

== system ErskineMultiDroneFormation/  Quadrotor2/Controller ==
  gyroscope : Inport
  attitude : Inport  Port=2
  velocity : Inport  Port=3
  position : Inport  Port=4
  input : Inport  Port=5
  Controller : MATLAB Function  TreatAsAtomicUnit=on
  Saturation : Saturate  UpperLimit=drone_params(DroneID).control.limits.thrust.max  LowerLimit=drone_params(DroneID).control.limits.thrust.min
  Saturation1 : Saturate  UpperLimit=0.1  LowerLimit=-0.1
  desired_prop_speed : MATLAB Function  TreatAsAtomicUnit=on
  prop_speeds : Outport
  wires:
  Controller/2(moments) -> Saturation1/1
  Saturation/1 -> desired_prop_speed/1(thrust)
  velocity/1 -> Controller/3(v)
  Saturation1/1 -> desired_prop_speed/2(moment)
  Controller/1(thrust) -> Saturation/1
  position/1 -> Controller/2(p)
  input/1 -> Controller/1(u)
  attitude/1 -> Controller/4(q)
  gyroscope/1 -> Controller/5(omega)
  desired_prop_speed/1(Omega_props) -> prop_speeds/1

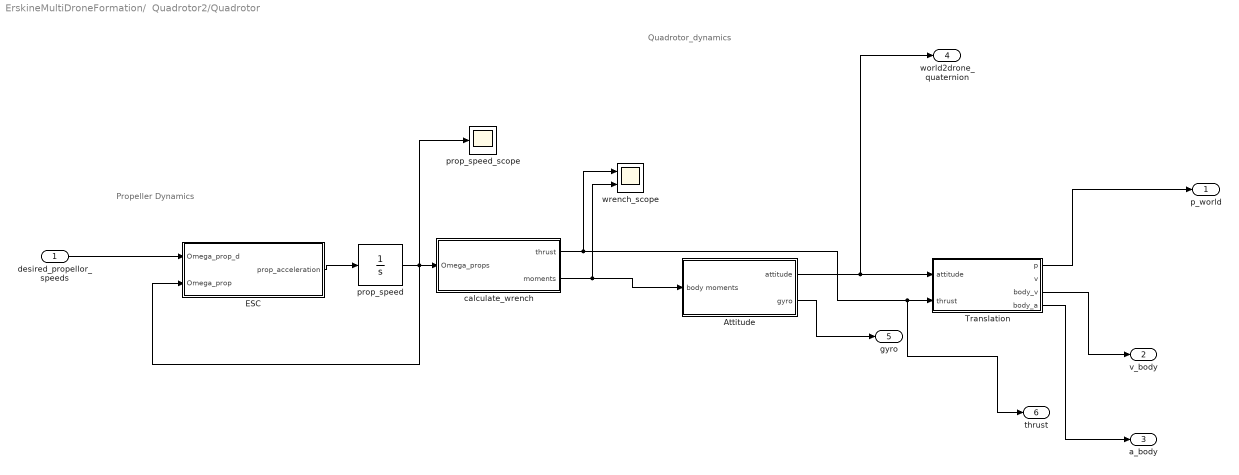
== system ErskineMultiDroneFormation/  Quadrotor2/Quadrotor ==
  note: Quadrotor_dynamics
  note: Propeller Dynamics
  desired_propellor_speeds : Inport
  Attitude : Subsystem
  ESC : MATLAB Function  TreatAsAtomicUnit=on
  Translation : Subsystem
  calculate_wrench : MATLAB Function  TreatAsAtomicUnit=on
  prop_speed : Integrator  InitialCondition=drone_params(DroneID).motors.omega0  LimitOutput=on  UpperSaturationLimit=drone_params(DroneID).motors.omega_max  LowerSaturationLimit=drone_params(DroneID).motors.omega_min
  prop_speed_scope : Scope
  wrench_scope : Scope  NumInputPorts=2
  p_world : Outport
  v_body : Outport  Port=2
  a_body : Outport  Port=3
  world2drone_quaternion : Outport  Port=4
  gyro : Outport  Port=5
  thrust : Outport  Port=6
  wires:
  calculate_wrench/1(thrust) -> wrench_scope/1, thrust/1, Translation/2(thrust)
  ESC/1(prop_acceleration) -> prop_speed/1
  desired_propellor_speeds/1 -> ESC/1(Omega_prop_d)
  prop_speed/1 -> prop_speed_scope/1, calculate_wrench/1(Omega_props), ESC/2(Omega_prop)
  calculate_wrench/2(moments) -> wrench_scope/2, Attitude/1(body moments)
  Attitude/1(attitude) -> world2drone_quaternion/1, Translation/1(attitude)
  Attitude/2(gyro) -> gyro/1
  Translation/3(body_v) -> v_body/1
  Translation/4(body_a) -> a_body/1
  Translation/1(p) -> p_world/1

== system ErskineMultiDroneFormation/  Quadrotor3/Controller ==
  gyroscope : Inport
  attitude : Inport  Port=2
  velocity : Inport  Port=3
  position : Inport  Port=4
  input : Inport  Port=5
  Controller : MATLAB Function  TreatAsAtomicUnit=on
  Saturation : Saturate  UpperLimit=16  LowerLimit=3
  Saturation1 : Saturate  UpperLimit=0.1  LowerLimit=-0.1
  desired_prop_speed : MATLAB Function  TreatAsAtomicUnit=on
  prop_speeds : Outport
  wires:
  Controller/2(moments) -> Saturation1/1
  Saturation/1 -> desired_prop_speed/1(thrust)
  velocity/1 -> Controller/3(v)
  Saturation1/1 -> desired_prop_speed/2(moment)
  Controller/1(thrust) -> Saturation/1
  position/1 -> Controller/2(p)
  input/1 -> Controller/1(u)
  attitude/1 -> Controller/4(q)
  gyroscope/1 -> Controller/5(omega)
  desired_prop_speed/1(Omega_props) -> prop_speeds/1

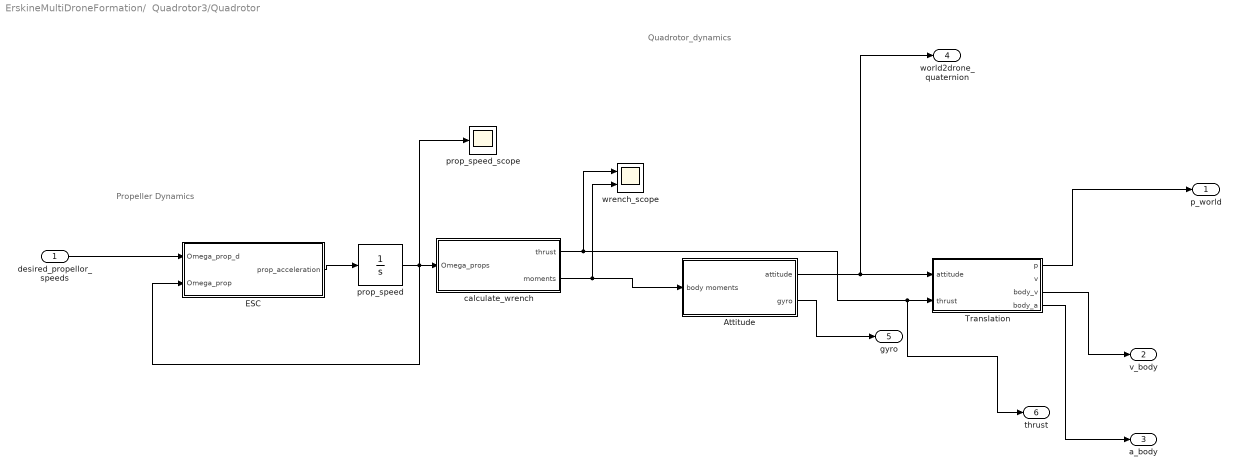
== system ErskineMultiDroneFormation/  Quadrotor3/Quadrotor ==
  note: Quadrotor_dynamics
  note: Propeller Dynamics
  desired_propellor_speeds : Inport
  Attitude : Subsystem
  ESC : MATLAB Function  TreatAsAtomicUnit=on
  Translation : Subsystem
  calculate_wrench : MATLAB Function  TreatAsAtomicUnit=on
  prop_speed : Integrator  InitialCondition=drone_params(DroneID).motors.omega0  LimitOutput=on  UpperSaturationLimit=drone_params(DroneID).motors.omega_max  LowerSaturationLimit=drone_params(DroneID).motors.omega_min
  prop_speed_scope : Scope
  wrench_scope : Scope  NumInputPorts=2
  p_world : Outport
  v_body : Outport  Port=2
  a_body : Outport  Port=3
  world2drone_quaternion : Outport  Port=4
  gyro : Outport  Port=5
  thrust : Outport  Port=6
  wires:
  calculate_wrench/1(thrust) -> wrench_scope/1, thrust/1, Translation/2(thrust)
  ESC/1(prop_acceleration) -> prop_speed/1
  desired_propellor_speeds/1 -> ESC/1(Omega_prop_d)
  prop_speed/1 -> prop_speed_scope/1, calculate_wrench/1(Omega_props), ESC/2(Omega_prop)
  calculate_wrench/2(moments) -> wrench_scope/2, Attitude/1(body moments)
  Attitude/1(attitude) -> world2drone_quaternion/1, Translation/1(attitude)
  Attitude/2(gyro) -> gyro/1
  Translation/3(body_v) -> v_body/1
  Translation/4(body_a) -> a_body/1
  Translation/1(p) -> p_world/1

== system ErskineMultiDroneFormation/  Quadrotor4/Controller ==
  gyroscope : Inport
  attitude : Inport  Port=2
  velocity : Inport  Port=3
  position : Inport  Port=4
  input : Inport  Port=5
  Controller : MATLAB Function  TreatAsAtomicUnit=on
  Saturation : Saturate  UpperLimit=drone_params(DroneID).control.limits.thrust.max  LowerLimit=drone_params(DroneID).control.limits.thrust.min
  Saturation1 : Saturate  UpperLimit=0.1  LowerLimit=-0.1
  desired_prop_speed : MATLAB Function  TreatAsAtomicUnit=on
  prop_speeds : Outport
  wires:
  Controller/2(moments) -> Saturation1/1
  Saturation/1 -> desired_prop_speed/1(thrust)
  velocity/1 -> Controller/3(v)
  Saturation1/1 -> desired_prop_speed/2(moment)
  Controller/1(thrust) -> Saturation/1
  position/1 -> Controller/2(p)
  input/1 -> Controller/1(u)
  attitude/1 -> Controller/4(q)
  gyroscope/1 -> Controller/5(omega)
  desired_prop_speed/1(Omega_props) -> prop_speeds/1

== system ErskineMultiDroneFormation/  Quadrotor4/Quadrotor ==
  note: Quadrotor_dynamics
  note: Propeller Dynamics
  desired_propellor_speeds : Inport
  Attitude : Subsystem
  ESC : MATLAB Function  TreatAsAtomicUnit=on
  Translation : Subsystem
  calculate_wrench : MATLAB Function  TreatAsAtomicUnit=on
  prop_speed : Integrator  InitialCondition=drone_params(DroneID).motors.omega0  LimitOutput=on  UpperSaturationLimit=drone_params(DroneID).motors.omega_max  LowerSaturationLimit=drone_params(DroneID).motors.omega_min
  prop_speed_scope : Scope
  wrench_scope : Scope  NumInputPorts=2
  p_world : Outport
  v_body : Outport  Port=2
  a_body : Outport  Port=3
  world2drone_quaternion : Outport  Port=4
  gyro : Outport  Port=5
  thrust : Outport  Port=6
  wires:
  calculate_wrench/1(thrust) -> wrench_scope/1, thrust/1, Translation/2(thrust)
  ESC/1(prop_acceleration) -> prop_speed/1
  desired_propellor_speeds/1 -> ESC/1(Omega_prop_d)
  prop_speed/1 -> prop_speed_scope/1, calculate_wrench/1(Omega_props), ESC/2(Omega_prop)
  calculate_wrench/2(moments) -> wrench_scope/2, Attitude/1(body moments)
  Attitude/1(attitude) -> world2drone_quaternion/1, Translation/1(attitude)
  Attitude/2(gyro) -> gyro/1
  Translation/3(body_v) -> v_body/1
  Translation/4(body_a) -> a_body/1
  Translation/1(p) -> p_world/1

== system ErskineMultiDroneFormation/  Quadrotor5/Controller ==
  gyroscope : Inport
  attitude : Inport  Port=2
  velocity : Inport  Port=3
  position : Inport  Port=4
  input : Inport  Port=5
  Controller : MATLAB Function  TreatAsAtomicUnit=on
  Saturation : Saturate  UpperLimit=drone_params(DroneID).control.limits.thrust.max  LowerLimit=drone_params(DroneID).control.limits.thrust.min
  Saturation1 : Saturate  UpperLimit=0.1  LowerLimit=-0.1
  desired_prop_speed : MATLAB Function  TreatAsAtomicUnit=on
  prop_speeds : Outport
  wires:
  Controller/2(moments) -> Saturation1/1
  Saturation/1 -> desired_prop_speed/1(thrust)
  velocity/1 -> Controller/3(v)
  Saturation1/1 -> desired_prop_speed/2(moment)
  Controller/1(thrust) -> Saturation/1
  position/1 -> Controller/2(p)
  input/1 -> Controller/1(u)
  attitude/1 -> Controller/4(q)
  gyroscope/1 -> Controller/5(omega)
  desired_prop_speed/1(Omega_props) -> prop_speeds/1

== system ErskineMultiDroneFormation/  Quadrotor5/Quadrotor ==
  note: Quadrotor_dynamics
  note: Propeller Dynamics
  desired_propellor_speeds : Inport
  Attitude : Subsystem
  ESC : MATLAB Function  TreatAsAtomicUnit=on
  Translation : Subsystem
  calculate_wrench : MATLAB Function  TreatAsAtomicUnit=on
  prop_speed : Integrator  InitialCondition=drone_params(DroneID).motors.omega0  LimitOutput=on  UpperSaturationLimit=drone_params(DroneID).motors.omega_max  LowerSaturationLimit=drone_params(DroneID).motors.omega_min
  prop_speed_scope : Scope
  wrench_scope : Scope  NumInputPorts=2
  p_world : Outport
  v_body : Outport  Port=2
  a_body : Outport  Port=3
  world2drone_quaternion : Outport  Port=4
  gyro : Outport  Port=5
  thrust : Outport  Port=6
  wires:
  calculate_wrench/1(thrust) -> wrench_scope/1, thrust/1, Translation/2(thrust)
  ESC/1(prop_acceleration) -> prop_speed/1
  desired_propellor_speeds/1 -> ESC/1(Omega_prop_d)
  prop_speed/1 -> prop_speed_scope/1, calculate_wrench/1(Omega_props), ESC/2(Omega_prop)
  calculate_wrench/2(moments) -> wrench_scope/2, Attitude/1(body moments)
  Attitude/1(attitude) -> world2drone_quaternion/1, Translation/1(attitude)
  Attitude/2(gyro) -> gyro/1
  Translation/3(body_v) -> v_body/1
  Translation/4(body_a) -> a_body/1
  Translation/1(p) -> p_world/1

== system ErskineMultiDroneFormation/  Quadrotor6/Controller ==
  gyroscope : Inport
  attitude : Inport  Port=2
  velocity : Inport  Port=3
  position : Inport  Port=4
  input : Inport  Port=5
  Controller : MATLAB Function  TreatAsAtomicUnit=on
  Saturation : Saturate  UpperLimit=16  LowerLimit=3
  Saturation1 : Saturate  UpperLimit=0.1  LowerLimit=-0.1
  desired_prop_speed : MATLAB Function  TreatAsAtomicUnit=on
  prop_speeds : Outport
  wires:
  Controller/2(moments) -> Saturation1/1
  Saturation/1 -> desired_prop_speed/1(thrust)
  velocity/1 -> Controller/3(v)
  Saturation1/1 -> desired_prop_speed/2(moment)
  Controller/1(thrust) -> Saturation/1
  position/1 -> Controller/2(p)
  input/1 -> Controller/1(u)
  attitude/1 -> Controller/4(q)
  gyroscope/1 -> Controller/5(omega)
  desired_prop_speed/1(Omega_props) -> prop_speeds/1

== system ErskineMultiDroneFormation/  Quadrotor6/Quadrotor ==
  note: Quadrotor_dynamics
  note: Propeller Dynamics
  desired_propellor_speeds : Inport
  Attitude : Subsystem
  ESC : MATLAB Function  TreatAsAtomicUnit=on
  Translation : Subsystem
  calculate_wrench : MATLAB Function  TreatAsAtomicUnit=on
  prop_speed : Integrator  InitialCondition=drone_params(DroneID).motors.omega0  LimitOutput=on  UpperSaturationLimit=drone_params(DroneID).motors.omega_max  LowerSaturationLimit=drone_params(DroneID).motors.omega_min
  prop_speed_scope : Scope
  wrench_scope : Scope  NumInputPorts=2
  p_world : Outport
  v_body : Outport  Port=2
  a_body : Outport  Port=3
  world2drone_quaternion : Outport  Port=4
  gyro : Outport  Port=5
  thrust : Outport  Port=6
  wires:
  calculate_wrench/1(thrust) -> wrench_scope/1, thrust/1, Translation/2(thrust)
  ESC/1(prop_acceleration) -> prop_speed/1
  desired_propellor_speeds/1 -> ESC/1(Omega_prop_d)
  prop_speed/1 -> prop_speed_scope/1, calculate_wrench/1(Omega_props), ESC/2(Omega_prop)
  calculate_wrench/2(moments) -> wrench_scope/2, Attitude/1(body moments)
  Attitude/1(attitude) -> world2drone_quaternion/1, Translation/1(attitude)
  Attitude/2(gyro) -> gyro/1
  Translation/3(body_v) -> v_body/1
  Translation/4(body_a) -> a_body/1
  Translation/1(p) -> p_world/1

== system ErskineMultiDroneFormation/  Quadrotor1/Quadrotor/Attitude ==
  body moments : Inport
  Attitude : Integrator  InitialCondition=q0(:,DroneID)
  MATLAB Function : MATLAB Function  TreatAsAtomicUnit=on
  MATLAB Function1 : MATLAB Function  TreatAsAtomicUnit=on
  Normalize Vector : vrlib/Utilities/Normalize Vector  maxzero=0
      settings: SourceProductName=Simulink
  Sine Wave : Sin  Commented=on  Amplitude=[0.5;0.5;0.5]  Frequency=[1;0.3;0.6]  SampleTime=0
  angular velocity : Integrator  InitialCondition=omega0(:,DroneID)
  attitude : Outport
  gyro : Outport  Port=2
  wires:
  Attitude/1 -> Normalize Vector/1
  MATLAB Function/1(qd) -> Attitude/1  "quaternion derivative"
  body moments/1 -> MATLAB Function1/1(m)
  MATLAB Function1/1(a) -> angular velocity/1  "body angular acceleration"
  angular velocity/1 -> gyro/1, MATLAB Function/2(omega), MATLAB Function1/2(omega)  "gyroscope"
  Normalize Vector/1 -> MATLAB Function/1(q), attitude/1  "unit quaternion"

== system ErskineMultiDroneFormation/  Quadrotor1/Quadrotor/Translation ==
  attitude : Inport
  thrust : Inport  Port=2
  MATLAB Function : MATLAB Function  TreatAsAtomicUnit=on
  MATLAB Function1 : MATLAB Function  TreatAsAtomicUnit=on
  Matrix Divide : Product  Inputs=/*  Multiplication=Matrix(*)
  Matrix Divide1 : Product  Inputs=/*  Multiplication=Matrix(*)
  position : Integrator  InitialCondition=p0(:,DroneID)
  velocity : Integrator  InitialCondition=v0(:,DroneID)
  p : Outport
  v : Outport  Port=2
  body_v : Outport  Port=3
  body_a : Outport  Port=4
  wires:
  velocity/1 -> Matrix Divide/2, v/1, position/1  "velocity"
  position/1 -> p/1  "position"
  MATLAB Function/1(a) -> Matrix Divide1/2, velocity/1  "acceleration"
  attitude/1 -> MATLAB Function1/1(q)
  thrust/1 -> MATLAB Function/1(f)
  MATLAB Function1/1(R) -> Matrix Divide1/1, Matrix Divide/1, MATLAB Function/2(R)
  Matrix Divide/1 -> body_v/1
  Matrix Divide1/1 -> body_a/1
